simulink model "robot_butaiguihua"  (R2019b)
settings: Solver=VariableStepAuto  StartTime=0.0  StopTime=80  RelTol=1e-3  EnableMultiTasking=on
undefined symbols (not defined in the file): X, Y, Z
libraries: sm_lib x54, nesl_utility x13, Contact_Forces_Lib x4, simulink_extras x4
(part 2 of 2)

== system robot_butaiguihua/BL/Subsystem5 ==
  File Solid3 : sm_lib/Body Elements/File Solid  ExtGeomFileName=E:\BaiduNetdiskDownload\dog_1\left_3.stl  UnitType=Custom  ExtGeomFileUnits=mm  StepReaderType=HEX  ExportEntireGeometry=off  InertiaType=CalculateFromGeometry  Mass=1  MassUnits=kg  CenterOfMass=[0 0 0]  CenterOfMassUnits=m  MomentsOfInertia=[1 1 1]  MomentsOfInertiaUnits=kg*m^2  ProductsOfInertia=[0 0 0]  ProductsOfInertiaUnits=kg*m^2  BasedOnType=Density  Density=1000  DensityUnits=kg/m^3  DoExposeReferenceFrame=on  SerializedFrames=<Frames/>  GraphicType=FromGeometry  MarkerShape=Sphere  MarkerSize=10  GraphicVisPropType=SimpleVisualProperties  GraphicDiffuseColor=[0.5 0.5 0.5]  GraphicSpecularColor=[0.5 0.5 0.5 1.0]  GraphicAmbientColor=[0.15 0.15 0.15 1.0]  GraphicEmissiveColor=[0.0 0.0 0.0 1.0]  GraphicShininess=75  GraphicOpacity=1.0
  Rigid Transform8 : sm_lib/Frames and Transforms/Rigid Transform  TranslationMethod=None  TranslationStandardOffset=0  TranslationLengthUnit=mm  TranslationStandardAxis=+Z  TranslationCartesianOffset=[27.5 0 -11.3]  TranslationROffset=0  TranslationROffsetUnits=m  TranslationZOffset=0  TranslationZOffsetUnits=m  TranslationThetaOffset=0  TranslationThetaOffsetUnits=deg  RotationMethod=StandardAxis  RotationAngleUnits=deg  RotationStandardAxis=+Z  RotationAngle=-90  RotationArbitraryAxis=[0 0 1]  FollAlignAxisA=+X  BaseAlignAxisA=+Y  FollAlignAxisB=+Y  BaseAlignAxisB=+Z  RotationSequenceAxes=FollowerAxes  RotationSequence=XYX  RotationSequenceAngles=[0 0 0]  RotationSequenceAnglesUnits=deg  RotationMatrix=[1 0 0; 0 1 0; 0 0 1]
  Rigid Transform9 : sm_lib/Frames and Transforms/Rigid Transform  TranslationMethod=Cartesian  TranslationStandardOffset=0  TranslationLengthUnit=mm  TranslationStandardAxis=+Z  TranslationCartesianOffset=[122.5 -2.5 0]  TranslationROffset=0  TranslationROffsetUnits=m  TranslationZOffset=0  TranslationZOffsetUnits=m  TranslationThetaOffset=0  TranslationThetaOffsetUnits=deg  RotationMethod=None  RotationAngleUnits=deg  RotationStandardAxis=+Y  RotationAngle=90  RotationArbitraryAxis=[0 0 1]  FollAlignAxisA=+X  BaseAlignAxisA=+Y  FollAlignAxisB=+Y  BaseAlignAxisB=+Z  RotationSequenceAxes=FollowerAxes  RotationSequence=XYX  RotationSequenceAngles=[0 0 0]  RotationSequenceAnglesUnits=deg  RotationMatrix=[1 0 0; 0 1 0; 0 0 1]
  Conn1 : PMIOPort  Side=Right
  Conn2 : PMIOPort  Port=2  Side=Left
  connections:
  Rigid Transform8/LConn1 -- Conn2/RConn1
  Rigid Transform9/RConn1 -- Conn1/RConn1
  File Solid3/RConn1 -- Rigid Transform8/RConn1 -- Rigid Transform9/LConn1

== system robot_butaiguihua/BR/Subsystem10 ==
  File Solid2 : sm_lib/Body Elements/File Solid  ExtGeomFileName=E:\BaiduNetdiskDownload\dog_1\right_2.stl  UnitType=Custom  ExtGeomFileUnits=mm  StepReaderType=HEX  ExportEntireGeometry=off  InertiaType=CalculateFromGeometry  Mass=1  MassUnits=kg  CenterOfMass=[0 0 0]  CenterOfMassUnits=m  MomentsOfInertia=[1 1 1]  MomentsOfInertiaUnits=kg*m^2  ProductsOfInertia=[0 0 0]  ProductsOfInertiaUnits=kg*m^2  BasedOnType=Density  Density=1000  DensityUnits=kg/m^3  DoExposeReferenceFrame=on  SerializedFrames=<Frames/>  GraphicType=FromGeometry  MarkerShape=Sphere  MarkerSize=10  GraphicVisPropType=SimpleVisualProperties  GraphicDiffuseColor=[0.5 0.5 0.5]  GraphicSpecularColor=[0.5 0.5 0.5 1.0]  GraphicAmbientColor=[0.15 0.15 0.15 1.0]  GraphicEmissiveColor=[0.0 0.0 0.0 1.0]  GraphicShininess=75  GraphicOpacity=1.0
  Rigid Transform7 : sm_lib/Frames and Transforms/Rigid Transform  TranslationMethod=Cartesian  TranslationStandardOffset=0  TranslationLengthUnit=mm  TranslationStandardAxis=+Z  TranslationCartesianOffset=[-14.5 -107.5 0]  TranslationROffset=0  TranslationROffsetUnits=m  TranslationZOffset=0  TranslationZOffsetUnits=m  TranslationThetaOffset=0  TranslationThetaOffsetUnits=deg  RotationMethod=None  RotationAngleUnits=deg  RotationStandardAxis=+Y  RotationAngle=90  RotationArbitraryAxis=[0 0 1]  FollAlignAxisA=+X  BaseAlignAxisA=+Y  FollAlignAxisB=+Y  BaseAlignAxisB=+Z  RotationSequenceAxes=FollowerAxes  RotationSequence=XYX  RotationSequenceAngles=[0 0 0]  RotationSequenceAnglesUnits=deg  RotationMatrix=[1 0 0; 0 1 0; 0 0 1]
  Conn1 : PMIOPort  Side=Left
  Conn2 : PMIOPort  Port=2  Side=Right
  connections:
  Rigid Transform7/LConn1 -- File Solid2/RConn1 -- Conn1/RConn1
  Conn2/RConn1 -- Rigid Transform7/RConn1

== system robot_butaiguihua/BR/Subsystem11 ==
  File Solid3 : sm_lib/Body Elements/File Solid  ExtGeomFileName=E:\BaiduNetdiskDownload\dog_1\right_3.stl  UnitType=Custom  ExtGeomFileUnits=mm  StepReaderType=HEX  ExportEntireGeometry=off  InertiaType=CalculateFromGeometry  Mass=1  MassUnits=kg  CenterOfMass=[0 0 0]  CenterOfMassUnits=m  MomentsOfInertia=[1 1 1]  MomentsOfInertiaUnits=kg*m^2  ProductsOfInertia=[0 0 0]  ProductsOfInertiaUnits=kg*m^2  BasedOnType=Density  Density=1000  DensityUnits=kg/m^3  DoExposeReferenceFrame=on  SerializedFrames=<Frames/>  GraphicType=FromGeometry  MarkerShape=Sphere  MarkerSize=10  GraphicVisPropType=SimpleVisualProperties  GraphicDiffuseColor=[0.5 0.5 0.5]  GraphicSpecularColor=[0.5 0.5 0.5 1.0]  GraphicAmbientColor=[0.15 0.15 0.15 1.0]  GraphicEmissiveColor=[0.0 0.0 0.0 1.0]  GraphicShininess=75  GraphicOpacity=1.0
  Rigid Transform8 : sm_lib/Frames and Transforms/Rigid Transform  TranslationMethod=None  TranslationStandardOffset=0  TranslationLengthUnit=mm  TranslationStandardAxis=+Z  TranslationCartesianOffset=[27.5 0 -11.3]  TranslationROffset=0  TranslationROffsetUnits=m  TranslationZOffset=0  TranslationZOffsetUnits=m  TranslationThetaOffset=0  TranslationThetaOffsetUnits=deg  RotationMethod=StandardAxis  RotationAngleUnits=deg  RotationStandardAxis=+Z  RotationAngle=-90  RotationArbitraryAxis=[0 0 1]  FollAlignAxisA=+X  BaseAlignAxisA=+Y  FollAlignAxisB=+Y  BaseAlignAxisB=+Z  RotationSequenceAxes=FollowerAxes  RotationSequence=XYX  RotationSequenceAngles=[0 0 0]  RotationSequenceAnglesUnits=deg  RotationMatrix=[1 0 0; 0 1 0; 0 0 1]
  Rigid Transform9 : sm_lib/Frames and Transforms/Rigid Transform  TranslationMethod=Cartesian  TranslationStandardOffset=0  TranslationLengthUnit=mm  TranslationStandardAxis=+Z  TranslationCartesianOffset=[122.5 -2.5 0]  TranslationROffset=0  TranslationROffsetUnits=m  TranslationZOffset=0  TranslationZOffsetUnits=m  TranslationThetaOffset=0  TranslationThetaOffsetUnits=deg  RotationMethod=None  RotationAngleUnits=deg  RotationStandardAxis=+Y  RotationAngle=90  RotationArbitraryAxis=[0 0 1]  FollAlignAxisA=+X  BaseAlignAxisA=+Y  FollAlignAxisB=+Y  BaseAlignAxisB=+Z  RotationSequenceAxes=FollowerAxes  RotationSequence=XYX  RotationSequenceAngles=[0 0 0]  RotationSequenceAnglesUnits=deg  RotationMatrix=[1 0 0; 0 1 0; 0 0 1]
  Conn1 : PMIOPort  Side=Right
  Conn2 : PMIOPort  Port=2  Side=Left
  connections:
  Rigid Transform9/LConn1 -- Rigid Transform8/RConn1 -- File Solid3/RConn1
  Rigid Transform9/RConn1 -- Conn1/RConn1
  Rigid Transform8/LConn1 -- Conn2/RConn1

== system robot_butaiguihua/BR/Subsystem9 ==
  File Solid1 : sm_lib/Body Elements/File Solid  ExtGeomFileName=E:\BaiduNetdiskDownload\dog_1\right_1.stl  UnitType=Custom  ExtGeomFileUnits=mm  StepReaderType=HEX  ExportEntireGeometry=off  InertiaType=CalculateFromGeometry  Mass=1  MassUnits=kg  CenterOfMass=[0 0 0]  CenterOfMassUnits=m  MomentsOfInertia=[1 1 1]  MomentsOfInertiaUnits=kg*m^2  ProductsOfInertia=[0 0 0]  ProductsOfInertiaUnits=kg*m^2  BasedOnType=Density  Density=1000  DensityUnits=kg/m^3  DoExposeReferenceFrame=on  SerializedFrames=<Frames/>  GraphicType=FromGeometry  MarkerShape=Sphere  MarkerSize=10  GraphicVisPropType=SimpleVisualProperties  GraphicDiffuseColor=[0.5 0.5 0.5]  GraphicSpecularColor=[0.5 0.5 0.5 1.0]  GraphicAmbientColor=[0.15 0.15 0.15 1.0]  GraphicEmissiveColor=[0.0 0.0 0.0 1.0]  GraphicShininess=75  GraphicOpacity=1.0
  Rigid Transform5 : sm_lib/Frames and Transforms/Rigid Transform  TranslationMethod=StandardAxis  TranslationStandardOffset=5  TranslationLengthUnit=mm  TranslationStandardAxis=+Z  TranslationCartesianOffset=[0 0 -39]  TranslationROffset=0  TranslationROffsetUnits=m  TranslationZOffset=0  TranslationZOffsetUnits=m  TranslationThetaOffset=0  TranslationThetaOffsetUnits=deg  RotationMethod=StandardAxis  RotationAngleUnits=deg  RotationStandardAxis=+X  RotationAngle=180  RotationArbitraryAxis=[0 0 1]  FollAlignAxisA=+X  BaseAlignAxisA=+Y  FollAlignAxisB=+Y  BaseAlignAxisB=+Z  RotationSequenceAxes=FollowerAxes  RotationSequence=XYX  RotationSequenceAngles=[0 0 0]  RotationSequenceAnglesUnits=deg  RotationMatrix=[1 0 0; 0 1 0; 0 0 1]
  Rigid Transform6 : sm_lib/Frames and Transforms/Rigid Transform  TranslationMethod=Cartesian  TranslationStandardOffset=0  TranslationLengthUnit=mm  TranslationStandardAxis=+Z  TranslationCartesianOffset=[-27.5 0 -11.3]  TranslationROffset=0  TranslationROffsetUnits=m  TranslationZOffset=0  TranslationZOffsetUnits=m  TranslationThetaOffset=0  TranslationThetaOffsetUnits=deg  RotationMethod=StandardAxis  RotationAngleUnits=deg  RotationStandardAxis=+Y  RotationAngle=90  RotationArbitraryAxis=[0 0 1]  FollAlignAxisA=+X  BaseAlignAxisA=+Y  FollAlignAxisB=+Y  BaseAlignAxisB=+Z  RotationSequenceAxes=FollowerAxes  RotationSequence=XYX  RotationSequenceAngles=[0 0 0]  RotationSequenceAnglesUnits=deg  RotationMatrix=[1 0 0; 0 1 0; 0 0 1]
  Conn1 : PMIOPort  Side=Left
  Conn2 : PMIOPort  Port=2  Side=Right
  connections:
  Rigid Transform5/RConn1 -- File Solid1/RConn1 -- Rigid Transform6/LConn1
  Conn1/RConn1 -- Rigid Transform5/LConn1
  Conn2/RConn1 -- Rigid Transform6/RConn1

== system robot_butaiguihua/FL/Subsystem ==
  File Solid1 : sm_lib/Body Elements/File Solid  ExtGeomFileName=E:\BaiduNetdiskDownload\dog_1\left_1.stl  UnitType=Custom  ExtGeomFileUnits=mm  StepReaderType=HEX  ExportEntireGeometry=off  InertiaType=CalculateFromGeometry  Mass=1  MassUnits=kg  CenterOfMass=[0 0 0]  CenterOfMassUnits=m  MomentsOfInertia=[1 1 1]  MomentsOfInertiaUnits=kg*m^2  ProductsOfInertia=[0 0 0]  ProductsOfInertiaUnits=kg*m^2  BasedOnType=Density  Density=1000  DensityUnits=kg/m^3  DoExposeReferenceFrame=on  SerializedFrames=<Frames/>  GraphicType=FromGeometry  MarkerShape=Sphere  MarkerSize=10  GraphicVisPropType=SimpleVisualProperties  GraphicDiffuseColor=[0.5 0.5 0.5]  GraphicSpecularColor=[0.5 0.5 0.5 1.0]  GraphicAmbientColor=[0.15 0.15 0.15 1.0]  GraphicEmissiveColor=[0.0 0.0 0.0 1.0]  GraphicShininess=75  GraphicOpacity=1.0
  Rigid Transform5 : sm_lib/Frames and Transforms/Rigid Transform  TranslationMethod=Cartesian  TranslationStandardOffset=0  TranslationLengthUnit=mm  TranslationStandardAxis=+Z  TranslationCartesianOffset=[0 0 -39]  TranslationROffset=0  TranslationROffsetUnits=m  TranslationZOffset=0  TranslationZOffsetUnits=m  TranslationThetaOffset=0  TranslationThetaOffsetUnits=deg  RotationMethod=StandardAxis  RotationAngleUnits=deg  RotationStandardAxis=+X  RotationAngle=180  RotationArbitraryAxis=[0 0 1]  FollAlignAxisA=+X  BaseAlignAxisA=+Y  FollAlignAxisB=+Y  BaseAlignAxisB=+Z  RotationSequenceAxes=FollowerAxes  RotationSequence=XYX  RotationSequenceAngles=[0 0 0]  RotationSequenceAnglesUnits=deg  RotationMatrix=[1 0 0; 0 1 0; 0 0 1]
  Rigid Transform6 : sm_lib/Frames and Transforms/Rigid Transform  TranslationMethod=Cartesian  TranslationStandardOffset=0  TranslationLengthUnit=mm  TranslationStandardAxis=+Z  TranslationCartesianOffset=[27.5 0 -11.3]  TranslationROffset=0  TranslationROffsetUnits=m  TranslationZOffset=0  TranslationZOffsetUnits=m  TranslationThetaOffset=0  TranslationThetaOffsetUnits=deg  RotationMethod=StandardAxis  RotationAngleUnits=deg  RotationStandardAxis=+Y  RotationAngle=90  RotationArbitraryAxis=[0 0 1]  FollAlignAxisA=+X  BaseAlignAxisA=+Y  FollAlignAxisB=+Y  BaseAlignAxisB=+Z  RotationSequenceAxes=FollowerAxes  RotationSequence=XYX  RotationSequenceAngles=[0 0 0]  RotationSequenceAnglesUnits=deg  RotationMatrix=[1 0 0; 0 1 0; 0 0 1]
  Conn1 : PMIOPort  Side=Left
  Conn2 : PMIOPort  Port=2  Side=Right
  connections:
  Rigid Transform5/RConn1 -- Rigid Transform6/LConn1 -- File Solid1/RConn1
  Conn1/RConn1 -- Rigid Transform5/LConn1
  Conn2/RConn1 -- Rigid Transform6/RConn1

== system robot_butaiguihua/FL/Subsystem1 ==
  File Solid2 : sm_lib/Body Elements/File Solid  ExtGeomFileName=E:\BaiduNetdiskDownload\dog_1\left_2.stl  UnitType=Custom  ExtGeomFileUnits=mm  StepReaderType=HEX  ExportEntireGeometry=off  InertiaType=CalculateFromGeometry  Mass=1  MassUnits=kg  CenterOfMass=[0 0 0]  CenterOfMassUnits=m  MomentsOfInertia=[1 1 1]  MomentsOfInertiaUnits=kg*m^2  ProductsOfInertia=[0 0 0]  ProductsOfInertiaUnits=kg*m^2  BasedOnType=Density  Density=1000  DensityUnits=kg/m^3  DoExposeReferenceFrame=on  SerializedFrames=<Frames/>  GraphicType=FromGeometry  MarkerShape=Sphere  MarkerSize=10  GraphicVisPropType=SimpleVisualProperties  GraphicDiffuseColor=[0.5 0.5 0.5]  GraphicSpecularColor=[0.5 0.5 0.5 1.0]  GraphicAmbientColor=[0.15 0.15 0.15 1.0]  GraphicEmissiveColor=[0.0 0.0 0.0 1.0]  GraphicShininess=75  GraphicOpacity=1.0
  Rigid Transform7 : sm_lib/Frames and Transforms/Rigid Transform  TranslationMethod=Cartesian  TranslationStandardOffset=0  TranslationLengthUnit=mm  TranslationStandardAxis=+Z  TranslationCartesianOffset=[-14.5 -107.5 0]  TranslationROffset=0  TranslationROffsetUnits=m  TranslationZOffset=0  TranslationZOffsetUnits=m  TranslationThetaOffset=0  TranslationThetaOffsetUnits=deg  RotationMethod=None  RotationAngleUnits=deg  RotationStandardAxis=+Y  RotationAngle=90  RotationArbitraryAxis=[0 0 1]  FollAlignAxisA=+X  BaseAlignAxisA=+Y  FollAlignAxisB=+Y  BaseAlignAxisB=+Z  RotationSequenceAxes=FollowerAxes  RotationSequence=XYX  RotationSequenceAngles=[0 0 0]  RotationSequenceAnglesUnits=deg  RotationMatrix=[1 0 0; 0 1 0; 0 0 1]
  Conn1 : PMIOPort  Side=Left
  Conn2 : PMIOPort  Port=2  Side=Right
  connections:
  Rigid Transform7/LConn1 -- Conn1/RConn1 -- File Solid2/RConn1
  Conn2/RConn1 -- Rigid Transform7/RConn1

== system robot_butaiguihua/FL/Subsystem2 ==
  File Solid3 : sm_lib/Body Elements/File Solid  ExtGeomFileName=E:\BaiduNetdiskDownload\dog_1\left_3.stl  UnitType=Custom  ExtGeomFileUnits=mm  StepReaderType=HEX  ExportEntireGeometry=off  InertiaType=CalculateFromGeometry  Mass=1  MassUnits=kg  CenterOfMass=[0 0 0]  CenterOfMassUnits=m  MomentsOfInertia=[1 1 1]  MomentsOfInertiaUnits=kg*m^2  ProductsOfInertia=[0 0 0]  ProductsOfInertiaUnits=kg*m^2  BasedOnType=Density  Density=1000  DensityUnits=kg/m^3  DoExposeReferenceFrame=on  SerializedFrames=<Frames/>  GraphicType=FromGeometry  MarkerShape=Sphere  MarkerSize=10  GraphicVisPropType=SimpleVisualProperties  GraphicDiffuseColor=[0.5 0.5 0.5]  GraphicSpecularColor=[0.5 0.5 0.5 1.0]  GraphicAmbientColor=[0.15 0.15 0.15 1.0]  GraphicEmissiveColor=[0.0 0.0 0.0 1.0]  GraphicShininess=75  GraphicOpacity=1.0
  Rigid Transform8 : sm_lib/Frames and Transforms/Rigid Transform  TranslationMethod=None  TranslationStandardOffset=0  TranslationLengthUnit=mm  TranslationStandardAxis=+Z  TranslationCartesianOffset=[27.5 0 -11.3]  TranslationROffset=0  TranslationROffsetUnits=m  TranslationZOffset=0  TranslationZOffsetUnits=m  TranslationThetaOffset=0  TranslationThetaOffsetUnits=deg  RotationMethod=StandardAxis  RotationAngleUnits=deg  RotationStandardAxis=+Z  RotationAngle=-90  RotationArbitraryAxis=[0 0 1]  FollAlignAxisA=+X  BaseAlignAxisA=+Y  FollAlignAxisB=+Y  BaseAlignAxisB=+Z  RotationSequenceAxes=FollowerAxes  RotationSequence=XYX  RotationSequenceAngles=[0 0 0]  RotationSequenceAnglesUnits=deg  RotationMatrix=[1 0 0; 0 1 0; 0 0 1]
  Rigid Transform9 : sm_lib/Frames and Transforms/Rigid Transform  TranslationMethod=Cartesian  TranslationStandardOffset=0  TranslationLengthUnit=mm  TranslationStandardAxis=+Z  TranslationCartesianOffset=[122.5 -2.5 0]  TranslationROffset=0  TranslationROffsetUnits=m  TranslationZOffset=0  TranslationZOffsetUnits=m  TranslationThetaOffset=0  TranslationThetaOffsetUnits=deg  RotationMethod=None  RotationAngleUnits=deg  RotationStandardAxis=+Y  RotationAngle=90  RotationArbitraryAxis=[0 0 1]  FollAlignAxisA=+X  BaseAlignAxisA=+Y  FollAlignAxisB=+Y  BaseAlignAxisB=+Z  RotationSequenceAxes=FollowerAxes  RotationSequence=XYX  RotationSequenceAngles=[0 0 0]  RotationSequenceAnglesUnits=deg  RotationMatrix=[1 0 0; 0 1 0; 0 0 1]
  Conn1 : PMIOPort  Side=Right
  Conn2 : PMIOPort  Port=2  Side=Left
  connections:
  Rigid Transform9/LConn1 -- File Solid3/RConn1 -- Rigid Transform8/RConn1
  Rigid Transform9/RConn1 -- Conn1/RConn1
  Rigid Transform8/LConn1 -- Conn2/RConn1

== system robot_butaiguihua/FR/Subsystem6 ==
  File Solid1 : sm_lib/Body Elements/File Solid  ExtGeomFileName=E:\BaiduNetdiskDownload\dog_1\right_1.stl  UnitType=Custom  ExtGeomFileUnits=mm  StepReaderType=HEX  ExportEntireGeometry=off  InertiaType=CalculateFromGeometry  Mass=1  MassUnits=kg  CenterOfMass=[0 0 0]  CenterOfMassUnits=m  MomentsOfInertia=[1 1 1]  MomentsOfInertiaUnits=kg*m^2  ProductsOfInertia=[0 0 0]  ProductsOfInertiaUnits=kg*m^2  BasedOnType=Density  Density=1000  DensityUnits=kg/m^3  DoExposeReferenceFrame=on  SerializedFrames=<Frames/>  GraphicType=FromGeometry  MarkerShape=Sphere  MarkerSize=10  GraphicVisPropType=SimpleVisualProperties  GraphicDiffuseColor=[0.5 0.5 0.5]  GraphicSpecularColor=[0.5 0.5 0.5 1.0]  GraphicAmbientColor=[0.15 0.15 0.15 1.0]  GraphicEmissiveColor=[0.0 0.0 0.0 1.0]  GraphicShininess=75  GraphicOpacity=1.0
  Rigid Transform5 : sm_lib/Frames and Transforms/Rigid Transform  TranslationMethod=StandardAxis  TranslationStandardOffset=-39  TranslationLengthUnit=mm  TranslationStandardAxis=+Z  TranslationCartesianOffset=[0 0 -39]  TranslationROffset=0  TranslationROffsetUnits=m  TranslationZOffset=0  TranslationZOffsetUnits=m  TranslationThetaOffset=0  TranslationThetaOffsetUnits=deg  RotationMethod=StandardAxis  RotationAngleUnits=deg  RotationStandardAxis=+X  RotationAngle=180  RotationArbitraryAxis=[0 0 1]  FollAlignAxisA=+X  BaseAlignAxisA=+Y  FollAlignAxisB=+Y  BaseAlignAxisB=+Z  RotationSequenceAxes=FollowerAxes  RotationSequence=XYX  RotationSequenceAngles=[0 0 0]  RotationSequenceAnglesUnits=deg  RotationMatrix=[1 0 0; 0 1 0; 0 0 1]
  Rigid Transform6 : sm_lib/Frames and Transforms/Rigid Transform  TranslationMethod=Cartesian  TranslationStandardOffset=0  TranslationLengthUnit=mm  TranslationStandardAxis=+Z  TranslationCartesianOffset=[-27.5 0 -11.3]  TranslationROffset=0  TranslationROffsetUnits=m  TranslationZOffset=0  TranslationZOffsetUnits=m  TranslationThetaOffset=0  TranslationThetaOffsetUnits=deg  RotationMethod=StandardAxis  RotationAngleUnits=deg  RotationStandardAxis=+Y  RotationAngle=90  RotationArbitraryAxis=[0 0 1]  FollAlignAxisA=+X  BaseAlignAxisA=+Y  FollAlignAxisB=+Y  BaseAlignAxisB=+Z  RotationSequenceAxes=FollowerAxes  RotationSequence=XYX  RotationSequenceAngles=[0 0 0]  RotationSequenceAnglesUnits=deg  RotationMatrix=[1 0 0; 0 1 0; 0 0 1]
  Conn1 : PMIOPort  Side=Left
  Conn2 : PMIOPort  Port=2  Side=Right
  connections:
  Conn2/RConn1 -- Rigid Transform6/RConn1
  Conn1/RConn1 -- Rigid Transform5/LConn1
  Rigid Transform6/LConn1 -- File Solid1/RConn1 -- Rigid Transform5/RConn1

== system robot_butaiguihua/FR/Subsystem7 ==
  File Solid2 : sm_lib/Body Elements/File Solid  ExtGeomFileName=E:\BaiduNetdiskDownload\dog_1\right_2.stl  UnitType=Custom  ExtGeomFileUnits=mm  StepReaderType=HEX  ExportEntireGeometry=off  InertiaType=CalculateFromGeometry  Mass=1  MassUnits=kg  CenterOfMass=[0 0 0]  CenterOfMassUnits=m  MomentsOfInertia=[1 1 1]  MomentsOfInertiaUnits=kg*m^2  ProductsOfInertia=[0 0 0]  ProductsOfInertiaUnits=kg*m^2  BasedOnType=Density  Density=1000  DensityUnits=kg/m^3  DoExposeReferenceFrame=on  SerializedFrames=<Frames/>  GraphicType=FromGeometry  MarkerShape=Sphere  MarkerSize=10  GraphicVisPropType=SimpleVisualProperties  GraphicDiffuseColor=[0.5 0.5 0.5]  GraphicSpecularColor=[0.5 0.5 0.5 1.0]  GraphicAmbientColor=[0.15 0.15 0.15 1.0]  GraphicEmissiveColor=[0.0 0.0 0.0 1.0]  GraphicShininess=75  GraphicOpacity=1.0
  Rigid Transform7 : sm_lib/Frames and Transforms/Rigid Transform  TranslationMethod=Cartesian  TranslationStandardOffset=0  TranslationLengthUnit=mm  TranslationStandardAxis=+Z  TranslationCartesianOffset=[-14.5 -107.5 0]  TranslationROffset=0  TranslationROffsetUnits=m  TranslationZOffset=0  TranslationZOffsetUnits=m  TranslationThetaOffset=0  TranslationThetaOffsetUnits=deg  RotationMethod=None  RotationAngleUnits=deg  RotationStandardAxis=+Y  RotationAngle=90  RotationArbitraryAxis=[0 0 1]  FollAlignAxisA=+X  BaseAlignAxisA=+Y  FollAlignAxisB=+Y  BaseAlignAxisB=+Z  RotationSequenceAxes=FollowerAxes  RotationSequence=XYX  RotationSequenceAngles=[0 0 0]  RotationSequenceAnglesUnits=deg  RotationMatrix=[1 0 0; 0 1 0; 0 0 1]
  Conn1 : PMIOPort  Side=Left
  Conn2 : PMIOPort  Port=2  Side=Right
  connections:
  Conn2/RConn1 -- Rigid Transform7/RConn1
  Conn1/RConn1 -- File Solid2/RConn1 -- Rigid Transform7/LConn1

== system robot_butaiguihua/FR/Subsystem8 ==
  File Solid3 : sm_lib/Body Elements/File Solid  ExtGeomFileName=E:\BaiduNetdiskDownload\dog_1\right_3.stl  UnitType=Custom  ExtGeomFileUnits=mm  StepReaderType=HEX  ExportEntireGeometry=off  InertiaType=CalculateFromGeometry  Mass=1  MassUnits=kg  CenterOfMass=[0 0 0]  CenterOfMassUnits=m  MomentsOfInertia=[1 1 1]  MomentsOfInertiaUnits=kg*m^2  ProductsOfInertia=[0 0 0]  ProductsOfInertiaUnits=kg*m^2  BasedOnType=Density  Density=1000  DensityUnits=kg/m^3  DoExposeReferenceFrame=on  SerializedFrames=<Frames/>  GraphicType=FromGeometry  MarkerShape=Sphere  MarkerSize=10  GraphicVisPropType=SimpleVisualProperties  GraphicDiffuseColor=[0.5 0.5 0.5]  GraphicSpecularColor=[0.5 0.5 0.5 1.0]  GraphicAmbientColor=[0.15 0.15 0.15 1.0]  GraphicEmissiveColor=[0.0 0.0 0.0 1.0]  GraphicShininess=75  GraphicOpacity=1.0
  Rigid Transform8 : sm_lib/Frames and Transforms/Rigid Transform  TranslationMethod=None  TranslationStandardOffset=0  TranslationLengthUnit=mm  TranslationStandardAxis=+Z  TranslationCartesianOffset=[27.5 0 -11.3]  TranslationROffset=0  TranslationROffsetUnits=m  TranslationZOffset=0  TranslationZOffsetUnits=m  TranslationThetaOffset=0  TranslationThetaOffsetUnits=deg  RotationMethod=StandardAxis  RotationAngleUnits=deg  RotationStandardAxis=+Z  RotationAngle=-90  RotationArbitraryAxis=[0 0 1]  FollAlignAxisA=+X  BaseAlignAxisA=+Y  FollAlignAxisB=+Y  BaseAlignAxisB=+Z  RotationSequenceAxes=FollowerAxes  RotationSequence=XYX  RotationSequenceAngles=[0 0 0]  RotationSequenceAnglesUnits=deg  RotationMatrix=[1 0 0; 0 1 0; 0 0 1]
  Rigid Transform9 : sm_lib/Frames and Transforms/Rigid Transform  TranslationMethod=Cartesian  TranslationStandardOffset=0  TranslationLengthUnit=mm  TranslationStandardAxis=+Z  TranslationCartesianOffset=[122.5 -2.5 0]  TranslationROffset=0  TranslationROffsetUnits=m  TranslationZOffset=0  TranslationZOffsetUnits=m  TranslationThetaOffset=0  TranslationThetaOffsetUnits=deg  RotationMethod=None  RotationAngleUnits=deg  RotationStandardAxis=+Y  RotationAngle=90  RotationArbitraryAxis=[0 0 1]  FollAlignAxisA=+X  BaseAlignAxisA=+Y  FollAlignAxisB=+Y  BaseAlignAxisB=+Z  RotationSequenceAxes=FollowerAxes  RotationSequence=XYX  RotationSequenceAngles=[0 0 0]  RotationSequenceAnglesUnits=deg  RotationMatrix=[1 0 0; 0 1 0; 0 0 1]
  Conn1 : PMIOPort  Side=Right
  Conn2 : PMIOPort  Port=2  Side=Left
  connections:
  Rigid Transform8/LConn1 -- Conn2/RConn1
  Rigid Transform9/RConn1 -- Conn1/RConn1
  File Solid3/RConn1 -- Rigid Transform8/RConn1 -- Rigid Transform9/LConn1

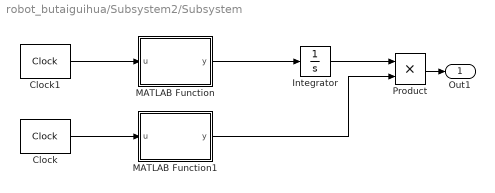
== system robot_butaiguihua/Subsystem2/Subsystem ==
  Clock : simulink_extras/Flip Flops/Clock  period=8
  Clock1 : simulink_extras/Flip Flops/Clock  period=4
  Integrator : Integrator
  MATLAB Function : MATLAB Function  TreatAsAtomicUnit=on
  MATLAB Function1 : MATLAB Function  TreatAsAtomicUnit=on
  Product : Product
  Out1 : Outport
  wires:
  MATLAB Function1/1(y) -> Product/2
  Clock/1 -> MATLAB Function1/1(u)
  Clock1/1 -> MATLAB Function/1(u)
  Product/1 -> Out1/1
  Integrator/1 -> Product/1
  MATLAB Function/1(y) -> Integrator/1

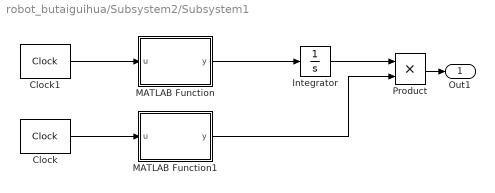
== system robot_butaiguihua/Subsystem2/Subsystem1 ==
  Clock : simulink_extras/Flip Flops/Clock  period=4
  Clock1 : simulink_extras/Flip Flops/Clock  period=2
  Integrator : Integrator
  MATLAB Function : MATLAB Function  TreatAsAtomicUnit=on
  MATLAB Function1 : MATLAB Function  TreatAsAtomicUnit=on
  Product : Product
  Out1 : Outport
  wires:
  Clock/1 -> MATLAB Function1/1(u)
  MATLAB Function/1(y) -> Integrator/1
  MATLAB Function1/1(y) -> Product/2
  Integrator/1 -> Product/1
  Product/1 -> Out1/1
  Clock1/1 -> MATLAB Function/1(u)

== matlab function robot_butaiguihua/Subsystem2/0-Tm-y1 ==
  data: u input; S input; y output; Tm input; H input
function y = fcn(u,S,Tm,H)

n=4;
if u>0
    y=2*H*(u/Tm-1/(n*pi)*sin(n*pi*u/Tm)).*(u>=0&u<Tm/2)+2*H*(1-u/Tm+1/(n*pi)*sin(n*pi*u/Tm)).*(u>=Tm/2&u<Tm);;
else 
    y=0;
end

== matlab function robot_butaiguihua/Subsystem2/0-Tm-x2 ==
  data: u input; Tm input; S input; x output
function x = fcn(u,Tm,S)

if u>0
    x =S*(u/Tm-1/(2*pi)*sin(2*pi*u/Tm));
else 
    u=-u;
     x =S*(u/Tm-1/(2*pi)*sin(2*pi*u/Tm));
end

== matlab function robot_butaiguihua/Subsystem2/0-Tm-x1 ==
  data: u input; x output; Tm input; S input
function x = fcn(u,Tm,S)


if u>0
   
    x =S*(u/Tm-1/(2*pi)*sin(2*pi*u/Tm));
else 
    u=-u;
    x =S*(u/Tm-1/(2*pi)*sin(2*pi*u/Tm));
end

== matlab function robot_butaiguihua/Subsystem2/0-Tm-y2 ==
  data: u input; S input; y output; Tm input; H input
function y = fcn(u,S,Tm,H)

n=4;
if u>0
    y=2*H*(u/Tm-1/(n*pi)*sin(n*pi*u/Tm)).*(u>=0&u<Tm/2)+2*H*(1-u/Tm+1/(n*pi)*sin(n*pi*u/Tm)).*(u>=Tm/2&u<Tm);;
else 
    y=0;
end

== matlab function robot_butaiguihua/Subsystem2/Subsystem/MATLAB Function ==
  data: u input; y output
function y = fcn(u)
if u==0
    y = -1;
else
    y=1;
end
end

== matlab function robot_butaiguihua/Subsystem2/Subsystem/MATLAB Function1 ==
  data: u input; y output
function y = fcn(u)
if u==0
    y = -1;
else
    y=1;
end
end

== matlab function robot_butaiguihua/Subsystem2/Subsystem1/MATLAB Function ==
  data: u input; y output
function y = fcn(u)
if u==0
    y = -1;
else
    y=1;
end
end

== matlab function robot_butaiguihua/Subsystem2/Subsystem1/MATLAB Function1 ==
  data: u input; y output
function y = fcn(u)
if u==0
    y = -1;
else
    y=1;
end
end

== matlab function robot_butaiguihua/逆运动学求解/MATLAB BR ==
  data: x input; alfa output; y input; z input; beta output; gamma output
function [alfa,beta,gamma]=xyztoang(x,y,z)
h=49.0;
hu=125.5899;
hl=116.0+20;

dyz=sqrt(y.^2+z.^2);
lyz=sqrt(dyz.^2-h.^2);
gamma_yz=-atan(y./z);
gamma_h_offset=-atan(h./lyz);
gamma=gamma_yz-gamma_h_offset;

lxzp=sqrt(lyz.^2+x.^2);
n=(lxzp.^2-hl^2-hu.^2)/(2*hu);
beta=-acos(n/hl);

alfa_xzp=-atan(x/lyz);
alfa_off=acos((hu+n)/lxzp);
alfa=(alfa_xzp+alfa_off);
end

== matlab function robot_butaiguihua/逆运动学求解/MATLAB BR1 ==
  data: x input; alfa output; y input; z input; beta output; gamma output
function [alfa,beta,gamma]=xyztoang(x,y,z)
h=49.0;
hu=125.5899;
hl=116.0+20;

dyz=sqrt(y.^2+z.^2);
lyz=sqrt(dyz.^2-h.^2);
gamma_yz=-atan(y./z);
gamma_h_offset=-atan(h./lyz);
gamma=gamma_yz-gamma_h_offset;

lxzp=sqrt(lyz.^2+x.^2);
n=(lxzp.^2-hl^2-hu.^2)/(2*hu);
beta=-acos(n/hl);

alfa_xzp=-atan(x/lyz);
alfa_off=acos((hu+n)/lxzp);
alfa=(alfa_xzp+alfa_off);
end

== matlab function robot_butaiguihua/逆运动学求解/MATLAB BR2 ==
  data: x input; alfa output; y input; z input; beta output; gamma output
function [alfa,beta,gamma]=xyztoang(x,y,z)
h=49.0;
hu=125.5899;
hl=116.0+20;

dyz=sqrt(y.^2+z.^2);
lyz=sqrt(dyz.^2-h.^2);
gamma_yz=-atan(y./z);
gamma_h_offset=-atan(h./lyz);
gamma=gamma_yz-gamma_h_offset;

lxzp=sqrt(lyz.^2+x.^2);
n=(lxzp.^2-hl^2-hu.^2)/(2*hu);
beta=-acos(n/hl);

alfa_xzp=-atan(x/lyz);
alfa_off=acos((hu+n)/lxzp);
alfa=(alfa_xzp+alfa_off);
end

== matlab function robot_butaiguihua/逆运动学求解/MATLAB BR3 ==
  data: x input; alfa output; y input; z input; beta output; gamma output
function [alfa,beta,gamma]=xyztoang(x,y,z)
h=49.0;
hu=125.5899;
hl=116.0+20;

dyz=sqrt(y.^2+z.^2);
lyz=sqrt(dyz.^2-h.^2);
gamma_yz=-atan(y./z);
gamma_h_offset=-atan(h./lyz);
gamma=gamma_yz-gamma_h_offset;

lxzp=sqrt(lyz.^2+x.^2);
n=(lxzp.^2-hl^2-hu.^2)/(2*hu);
beta=-acos(n/hl);

alfa_xzp=-atan(x/lyz);
alfa_off=acos((hu+n)/lxzp);
alfa=(alfa_xzp+alfa_off);
end
